simulink model "sliding_controller2"  (R2021a)
settings: Solver=ode3  StartTime=0.0  StopTime=inf  FixedStep=.001  RelTol=1e-3  EnableMultiTasking=on
model workspace (MAT data in the model file):
  SL_ROS_VariableLengthArrays_MaxSizes.CommonInfo.ArrayTruncateAction = 'EmitWarning'
  SL_ROS_VariableLengthArrays_MaxSizes.MsgTypeMap = containers.Map
  SL_ROS_VariableLengthArrays_MaxSizes.MsgTypeMap.serialization.keys = {'ambf_walker/DesiredJoints', 'rbdl_server/RBDLInverseDynamicsRequest', 'rbdl_server/RBDLInverseDynamicsResponse', 'sensor_msgs/JointState', 'std_msgs/Float32MultiArray', 'std_msgs/Float64MultiArray'}
  SL_ROS_VariableLengthArrays_MaxSizes.MsgTypeMap.serialization.values{1}(1).PropertyName = 'Controller'
  SL_ROS_VariableLengthArrays_MaxSizes.MsgTypeMap.serialization.values{1}(1).DataType = 'uint8'
  SL_ROS_VariableLengthArrays_MaxSizes.MsgTypeMap.serialization.values{1}(1).MaxLength = 8
  SL_ROS_VariableLengthArrays_MaxSizes.MsgTypeMap.serialization.values{1}(2).PropertyName = 'Other'
  SL_ROS_VariableLengthArrays_MaxSizes.MsgTypeMap.serialization.values{1}(2).DataType = 'double'
  SL_ROS_VariableLengthArrays_MaxSizes.MsgTypeMap.serialization.values{1}(2).MaxLength = 7
  SL_ROS_VariableLengthArrays_MaxSizes.MsgTypeMap.serialization.values{1}(3).PropertyName = 'Q'
  SL_ROS_VariableLengthArrays_MaxSizes.MsgTypeMap.serialization.values{1}(3).DataType = 'double'
  SL_ROS_VariableLengthArrays_MaxSizes.MsgTypeMap.serialization.values{1}(3).MaxLength = 7
  SL_ROS_VariableLengthArrays_MaxSizes.MsgTypeMap.serialization.values{1}(4).PropertyName = 'Qd'
  SL_ROS_VariableLengthArrays_MaxSizes.MsgTypeMap.serialization.values{1}(4).DataType = 'double'
  SL_ROS_VariableLengthArrays_MaxSizes.MsgTypeMap.serialization.values{1}(4).MaxLength = 7
  SL_ROS_VariableLengthArrays_MaxSizes.MsgTypeMap.serialization.values{1}(5).PropertyName = 'Qdd'
  SL_ROS_VariableLengthArrays_MaxSizes.MsgTypeMap.serialization.values{1}(5).DataType = 'double'
  SL_ROS_VariableLengthArrays_MaxSizes.MsgTypeMap.serialization.values{1}(5).MaxLength = 7
  SL_ROS_VariableLengthArrays_MaxSizes.MsgTypeMap.serialization.values{2}(1).PropertyName = 'ModelName'
  SL_ROS_VariableLengthArrays_MaxSizes.MsgTypeMap.serialization.values{2}(1).DataType = 'uint8'
  SL_ROS_VariableLengthArrays_MaxSizes.MsgTypeMap.serialization.values{2}(1).MaxLength = 4
  SL_ROS_VariableLengthArrays_MaxSizes.MsgTypeMap.serialization.values{2}(2).PropertyName = 'Q'
  SL_ROS_VariableLengthArrays_MaxSizes.MsgTypeMap.serialization.values{2}(2).DataType = 'double'
  SL_ROS_VariableLengthArrays_MaxSizes.MsgTypeMap.serialization.values{2}(2).MaxLength = 7
  SL_ROS_VariableLengthArrays_MaxSizes.MsgTypeMap.serialization.values{2}(3).PropertyName = 'Qd'
  SL_ROS_VariableLengthArrays_MaxSizes.MsgTypeMap.serialization.values{2}(3).DataType = 'double'
  SL_ROS_VariableLengthArrays_MaxSizes.MsgTypeMap.serialization.values{2}(3).MaxLength = 7
  SL_ROS_VariableLengthArrays_MaxSizes.MsgTypeMap.serialization.values{2}(4).PropertyName = 'Qdd'
  SL_ROS_VariableLengthArrays_MaxSizes.MsgTypeMap.serialization.values{2}(4).DataType = 'double'
  SL_ROS_VariableLengthArrays_MaxSizes.MsgTypeMap.serialization.values{2}(4).MaxLength = 7
  SL_ROS_VariableLengthArrays_MaxSizes.MsgTypeMap.serialization.values{3}.PropertyName = 'Tau'
  SL_ROS_VariableLengthArrays_MaxSizes.MsgTypeMap.serialization.values{3}.DataType = 'double'
  SL_ROS_VariableLengthArrays_MaxSizes.MsgTypeMap.serialization.values{3}.MaxLength = 7
  SL_ROS_VariableLengthArrays_MaxSizes.MsgTypeMap.serialization.values{4}(1).PropertyName = 'Effort'
  SL_ROS_VariableLengthArrays_MaxSizes.MsgTypeMap.serialization.values{4}(1).DataType = 'double'
  SL_ROS_VariableLengthArrays_MaxSizes.MsgTypeMap.serialization.values{4}(1).MaxLength = 7
  SL_ROS_VariableLengthArrays_MaxSizes.MsgTypeMap.serialization.values{4}(2).PropertyName = 'Name'
  SL_ROS_VariableLengthArrays_MaxSizes.MsgTypeMap.serialization.values{4}(2).DataType = 'std_msgs/String'
  SL_ROS_VariableLengthArrays_MaxSizes.MsgTypeMap.serialization.values{4}(2).MaxLength = 16
  SL_ROS_VariableLengthArrays_MaxSizes.MsgTypeMap.serialization.values{4}(3).PropertyName = 'Position'
  SL_ROS_VariableLengthArrays_MaxSizes.MsgTypeMap.serialization.values{4}(3).DataType = 'double'
  SL_ROS_VariableLengthArrays_MaxSizes.MsgTypeMap.serialization.values{4}(3).MaxLength = 7
  SL_ROS_VariableLengthArrays_MaxSizes.MsgTypeMap.serialization.values{4}(4).PropertyName = 'Velocity'
  SL_ROS_VariableLengthArrays_MaxSizes.MsgTypeMap.serialization.values{4}(4).DataType = 'double'
  SL_ROS_VariableLengthArrays_MaxSizes.MsgTypeMap.serialization.values{4}(4).MaxLength = 7
  SL_ROS_VariableLengthArrays_MaxSizes.MsgTypeMap.serialization.values{5}.PropertyName = 'Data'
  SL_ROS_VariableLengthArrays_MaxSizes.MsgTypeMap.serialization.values{5}.DataType = 'single'
  SL_ROS_VariableLengthArrays_MaxSizes.MsgTypeMap.serialization.values{5}.MaxLength = 7
  SL_ROS_VariableLengthArrays_MaxSizes.MsgTypeMap.serialization.values{6}.PropertyName = 'Data'
  SL_ROS_VariableLengthArrays_MaxSizes.MsgTypeMap.serialization.values{6}.DataType = 'double'
  SL_ROS_VariableLengthArrays_MaxSizes.MsgTypeMap.serialization.values{6}.MaxLength = 7
  SL_ROS_VariableLengthArrays_MaxSizes.MsgTypeMap.serialization.uniformity = 0
  SL_ROS_VariableLengthArrays_MaxSizes.MsgTypeMap.serialization.keyType = 'char'
  SL_ROS_VariableLengthArrays_MaxSizes.MsgTypeMap.serialization.valueType = 'any'
values from neighbouring files (symbols this model uses):
  alpha = [15,15]    [init_with_opt_gains.m]    (also in trying01.m = params.all_cost_parameters(5,1).Value; trying02.m = params.all_cost_parameters(5,1).Value)
  beta = zeros(7,1) + params.all_cost_parameters(6,1).Value(1)    [init_with_opt_gains.m]    (also in trying01.m; trying02.m = zeros(6,1) + params.all_cost_parameters(6,1).Value(1))
  Bn0 = [Bn0_hip Bn0_knee Bn0_ankle Bn0_hip Bn0_knee Bn0_ankle 0.0]    [init_with_opt_gains.m]    (also in sliding_controller_init.m = 50; trying01.m; trying02.m = [Bn0_hip Bn0_knee Bn0_ankle Bn0_hip Bn0_knee Bn0_ankle ])
  Bp0 = [Bp0_hip Bp0_knee Bp0_ankle Bp0_hip Bp0_knee Bp0_ankle 0.0]    [init_with_opt_gains.m]    (also in sliding_controller_init.m = 50; trying01.m; trying02.m = [Bp0_hip Bp0_knee Bp0_ankle Bp0_hip Bp0_knee Bp0_ankle ])
  dampener = 0.01*eye(2)    [init_with_opt_gains.m]    (also in sliding_controller_init.m = 100*eye(2); trying01.m = [30, 0; 0, 30]; trying02.m = [0.30, 0; 0, 0.30])
  Dm1 = 30*eye(7)    [init_with_opt_gains.m]    (also in sliding_controller_init.m; trying01.m = [Dm_hip, 0.0, 0.0, 0.0, 0.0, 0.0,0; trying02.m = [101.7013888888889 0 0 0 0 0)
  exo_sat = 150    [init_with_opt_gains.m]    (also in sliding_controller_init.m = 50; trying01.m = 250; trying02.m = 30)
  gamma = [15,15]    [init_with_opt_gains.m]    (also in trying01.m = params.all_cost_parameters(7,1).Value; trying02.m = params.all_cost_parameters(7,1).Value)
  human_sat = 30    [init_with_opt_gains.m]    (also in sliding_controller_init.m = 10; trying01.m = 0; trying02.m = 20)
  invMd = inv(Md)    [init_with_opt_gains.m]    (also in sliding_controller_init.m; trying01.m; trying02.m)
  Km1 = 30*eye(7)    [init_with_opt_gains.m]    (also in sliding_controller_init.m; trying01.m = [Km_hip, 0.0, 0.0, 0.0, 0.0, 0.0,0; trying02.m = [6120.116528948097 0 0 0 0 0)
  Kn0 = [Kn0_hip Kn0_knee Kn0_ankle Kn0_hip Kn0_knee Kn0_ankle 0.0]    [init_with_opt_gains.m]    (also in sliding_controller_init.m = 50*eye(7); trying01.m; trying02.m = [Kn0_hip Kn0_knee Kn0_ankle Kn0_hip Kn0_knee Kn0_ankle ])
  Kp0 = [Kp0_hip Kp0_knee Kp_ankle Kp0_hip Kp0_knee Kp0_ankle 0.0]    [init_with_opt_gains.m]    (also in sliding_controller_init.m = 50*eye(7); trying01.m = [Kp0_hip Kp0_knee Kp0_ankle Kp0_hip Kp0_knee Kp0_ankle 0.0]; trying02.m = [Kp0_hip Kp0_knee Kp0_ankle Kp0_hip Kp0_knee Kp0_ankle ])
  lambda2 = [lambda_hip, 0, 0, 0, 0, 0,0 ... (first row only)    [init_with_opt_gains.m]    (also in sliding_controller_init.m = eye(7); trying01.m; trying02.m = [lambda_hip, 0, 0, 0, 0, 0)
  rho2 = [rho_hip, 0.0, 0.0, 0.0, 0.0, 0.0,0 ... (first row only)    [init_with_opt_gains.m]    (also in sliding_controller_init.m = 200*eye(7); trying01.m; trying02.m = [rho_hip, 0.0, 0.0, 0.0, 0.0, 0.0)
  spring = 0.01*eye(2)    [init_with_opt_gains.m]    (also in sliding_controller_init.m = 100*eye(2); trying01.m = [30, 0; 0, 30]; trying02.m = [0.30, 0; 0, 0.30])
undefined symbols (not defined in the file or in its folder): Effort, Header, l, mh, Position, Q, Qd, Qdd, Velocity
libraries: robotlib x24
settings Model: SimulationMode=external  TunableVars=Bd,Bn0,Bp0,Dm1,Kd,Kd_e,Ked,Kem,Km1,Kn0,Kp0,Kp_e,Md,alpha_n,alpha_p,beta_n,beta_p,dampener,exo_sat,invMd,l1,l2,lambda2,myQ,myR,rho2,sat,spring  TunableVarsStorageClass=ExportedGlobal,ExportedGlobal,ExportedGlobal,ExportedGlobal,ExportedGlobal,ExportedGlobal,ExportedGlobal,ExportedGlobal,ExportedGlobal,ExportedGlobal,ExportedGlobal,ExportedGlobal,ExportedGlobal,ExportedGlobal,ExportedGlobal,ExportedGlobal,ExportedGlobal,ExportedGlobal,ExportedGlobal,ExportedGlobal,ExportedGlobal,ExportedGlobal,ExportedGlobal,ExportedGlobal,ExportedGlobal,ExportedGlobal,Auto,Auto  TunableVarsTypeQualifier=,,,,,,,,,,,,,,,,,,,,,,,,,,,  Creator=nathanielgoldfarb  LastModifiedBy=nathanielgoldfarb
settings OptimizationCC: EnhancedBackFolding=on  PassReuseOutputArgsAs=Individual arguments  ZeroExternalMemoryAtStartup=off  ZeroInternalMemoryAtStartup=off  InitFltsAndDblsToZero=on  MaxStackSize=64  OptimizeBlockOrder=speed  DifferentSizesBufferReuse=on  OptimizationCustomize=off  EfficientTunableParamExpr=on
settings DebuggingCC: ParameterTunabilityLossMsg=error
settings HardwareCC: ProdBitPerPointer=32  ProdBitPerSizeT=32  ProdBitPerPtrDiffT=32  ProdLargestAtomicFloat=None  ProdIntDivRoundTo=Undefined  ProdEndianess=Unspecified  ProdWordSize=32  ProdHWDeviceType=Generic->Unspecified (assume 32-bit Generic)  TargetLongLongMode=on
settings SFSimCC: MATLABDynamicMemAlloc=off  SimTargetLang=C++  GPUAcceleration=on  SimDLTargetLibrary=cudnn
settings RTWCC: SystemTargetFile=ert.tlc  HardwareBoard=Robot Operating System (ROS)  TLCOptions="-aInlineSetEventsForThisBaseRateFcn=TLC_FALSE -aSuppressMultiTaskScheduler=TLC_FALSE  -aRateBasedStepFcn=0"  TemplateMakefile=ert_default_tmf  GenerateReport=on  Toolchain=Catkin  LaunchReport=on  TargetLang=C++  GenerateCodeMetricsReport=on
settings CodeAppCC: ForceParamTrailComments=on  IgnoreCustomStorageClasses=off  OperatorAnnotations=on  SimulinkDataObjDesc=on  SFDataObjDesc=on  InsertBlockDesc=on
settings ERTTargetCC: CodeInterfacePackaging=C++ class  SupportContinuousTime=on  SupportNonInlinedSFcns=on  SupportVariableSizeSignals=on  RootIOFormat=Structure reference

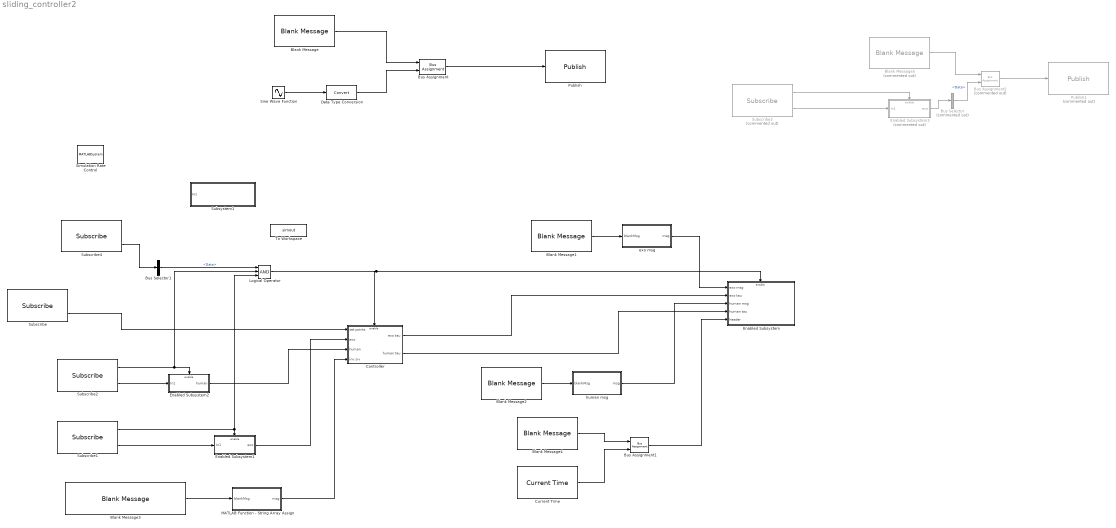
== system sliding_controller2 ==
  Blank Message : robotlib/Blank Message  messageClass=Message  entityType=std_msgs/Float32  messageType=std_msgs/Float32  SampleTime=-1  legacyBusStruct=off
  Blank Message1 : robotlib/Blank Message  messageClass=Message  entityType=sensor_msgs/JointState  messageType=sensor_msgs/JointState  SampleTime=inf  legacyBusStruct=off
  Blank Message2 : robotlib/Blank Message  messageClass=Message  entityType=sensor_msgs/JointState  messageType=sensor_msgs/JointState  SampleTime=inf  legacyBusStruct=off
  Blank Message3 : robotlib/Blank Message  messageClass=Service Request  entityType=rbdl_server/RBDLInverseDynamics  messageType=rbdl_server/RBDLInverseDynamicsRequest  SampleTime=inf  legacyBusStruct=off
  Blank Message4 : robotlib/Blank Message  messageClass=Message  entityType=std_msgs/Header  messageType=std_msgs/Header  SampleTime=inf  legacyBusStruct=off
  Blank Message5 : robotlib/Blank Message  Commented=on  messageClass=Message  entityType=std_msgs/Bool  messageType=std_msgs/Bool  SampleTime=inf  legacyBusStruct=off
  Bus Assignment : BusAssignment  AssignedSignals=Data
  Bus Assignment1 : BusAssignment  AssignedSignals=Stamp
  Bus Assignment2 : BusAssignment  Commented=on  AssignedSignals=Data
  Bus Selector : BusSelector  Commented=on  OutputSignals=Data
  Bus Selector1 : BusSelector  OutputSignals=Data
  Controller : Subsystem  TreatAsAtomicUnit=on
  Current Time : robotlib/Current Time  OutputFormat=bus  SampleTime=-1  ModelName=sliding_controller2
      settings: SourceProductBaseCode=RR
  Data Type Conversion : DataTypeConversion
  Enabled Subsystem : Subsystem  TreatAsAtomicUnit=on
  Enabled Subsystem1 : Subsystem  TreatAsAtomicUnit=on
  Enabled Subsystem2 : Subsystem  TreatAsAtomicUnit=on
  Enabled Subsystem3 : Subsystem  Commented=on  TreatAsAtomicUnit=on
  Logical Operator : Logic  Inputs=3  AllPortsSameDT=off  OutDataTypeStr=boolean
  MATLAB Function - String Array Assign : MATLAB Function  TreatAsAtomicUnit=on
  Publish : robotlib/Publish  topicSource=Specify your own  topic=/sin_wave  messageType=std_msgs/Float32  legacyBusStruct=off  messageQueueLength=1
  Publish1 : robotlib/Publish  Commented=on  topicSource=Specify your own  topic=/my_topic  messageType=std_msgs/Bool  legacyBusStruct=off  messageQueueLength=1
  Simulation Rate Control : MATLABSystem  System=ExampleHelperSimulationRateControl  SampleTime=0.001
      mask Type: ExampleHelperSimulationRateControl
      mask Display:
      | disp('Rate Control');
      | port_label('output',1,'r');
  Sine Wave Function : Sin  SampleTime=0
  Subscribe : robotlib/Subscribe  topicSource=Select from ROS network  topic=/exosimulink_set_points  messageType=ambf_walker/DesiredJoints  SampleTime=-1  legacyBusStruct=off  messageQueueLength=1
  Subscribe1 : robotlib/Subscribe  topicSource=Select from ROS network  topic=/exo_jointstate  messageType=sensor_msgs/JointState  SampleTime=-1  legacyBusStruct=off  messageQueueLength=1
  Subscribe2 : robotlib/Subscribe  topicSource=Select from ROS network  topic=/human_jointstate  messageType=sensor_msgs/JointState  SampleTime=-1  legacyBusStruct=off  messageQueueLength=1
  Subscribe3 : robotlib/Subscribe  Commented=on  topicSource=Specify your own  topic=/start  messageType=std_msgs/Bool  SampleTime=-1  legacyBusStruct=off  messageQueueLength=1
  Subscribe4 : robotlib/Subscribe  topicSource=Specify your own  topic=/start_sim  messageType=std_msgs/Bool  SampleTime=-1  legacyBusStruct=off  messageQueueLength=1
  Subsystem1 : Subsystem
  To Workspace : ToWorkspace  VariableName=simout  SampleTime=-1
      settings: Save2DSignal=2-D array (concatenate along first dimension)
  exo msg : MATLAB Function  TreatAsAtomicUnit=on
  human msg : MATLAB Function  TreatAsAtomicUnit=on
  wires:
  Data Type Conversion/1 -> Bus Assignment/2
  Blank Message/1 -> Bus Assignment/1
  Sine Wave Function/1 -> Data Type Conversion/1
  Bus Assignment/1 -> Publish/1
  human msg/1(msg) -> Enabled Subsystem/3(human msg)
  Controller/1(exo tau) -> Enabled Subsystem/2(exo tau)
  Blank Message2/1 -> human msg/1(blankMsg)
  Enabled Subsystem2/1(human) -> Controller/3(human)
  Blank Message1/1 -> exo msg/1(blankMsg)
  MATLAB Function - String Array Assign/1(msg) -> Controller/4(inv srv)
  Blank Message3/1 -> MATLAB Function - String Array Assign/1(blankMsg)
  Controller/2(human tau) -> Enabled Subsystem/4(human tau)
  Subscribe2/2 -> Enabled Subsystem2/1(In1)
  Subscribe1/2 -> Enabled Subsystem1/1(In1)
  Enabled Subsystem1/1(exo) -> Controller/2(exo)
  exo msg/1(msg) -> Enabled Subsystem/1(exo msg)
  Subscribe2/1 -> Logical Operator/2, Enabled Subsystem2/Enable
  Subscribe1/1 -> Enabled Subsystem1/Enable, Logical Operator/3
  Blank Message4/1 -> Bus Assignment1/1
  Current Time/1 -> Bus Assignment1/2
  Bus Assignment1/1 -> Enabled Subsystem/5(header)
  Subscribe3/2 -> Enabled Subsystem3/1(In1)
  Subscribe3/1 -> Enabled Subsystem3/Enable
  Enabled Subsystem3/1(exo) -> Bus Selector/1
  Bus Selector/1 -> Bus Assignment2/2  "<Data>"
  Blank Message5/1 -> Bus Assignment2/1
  Bus Assignment2/1 -> Publish1/1
  Subscribe4/2 -> Bus Selector1/1
  Bus Selector1/1 -> Logical Operator/1  "<Data>"
  Logical Operator/1 -> Enabled Subsystem/Enable, Controller/Enable
  Subscribe/2 -> Controller/1(set points)

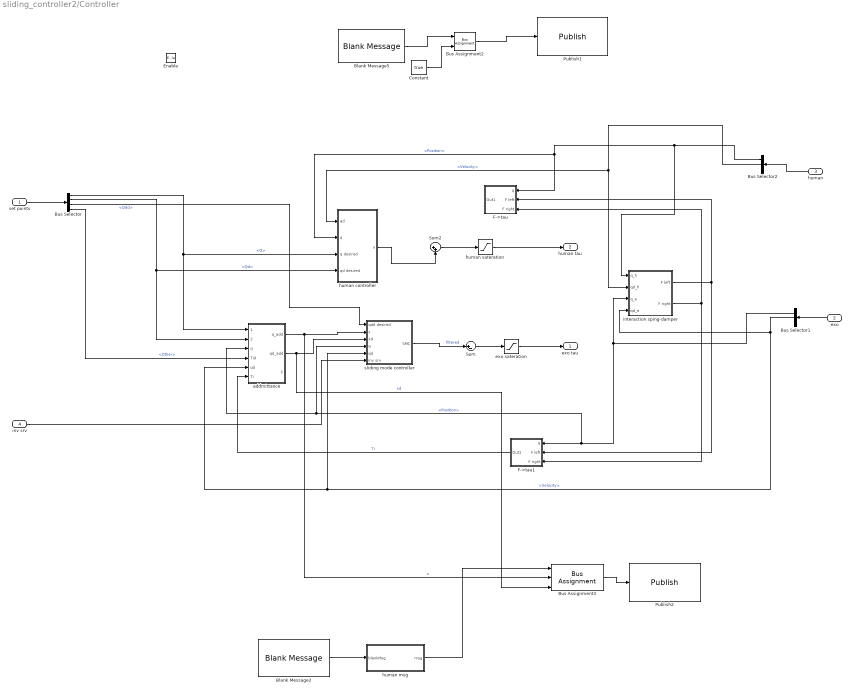
== system sliding_controller2/Controller ==
  set points : Inport
  exo : Inport  Port=2
  human : Inport  Port=3
  inv srv : Inport  Port=4
  Enable : EnablePort
  " interaction sping-damper" : Subsystem
  Blank Message2 : robotlib/Blank Message  messageClass=Message  entityType=sensor_msgs/JointState  messageType=sensor_msgs/JointState  SampleTime=inf  legacyBusStruct=off
  Blank Message5 : robotlib/Blank Message  messageClass=Message  entityType=std_msgs/Bool  messageType=std_msgs/Bool  SampleTime=inf  legacyBusStruct=off
  Bus Assignment2 : BusAssignment  AssignedSignals=Data
  Bus Assignment3 : BusAssignment  AssignedSignals=Position,Velocity
  Bus Selector : BusSelector  OutputSignals=Q,Qd,Qdd,Other
  Bus Selector1 : BusSelector  OutputSignals=Position,Velocity,Effort
  Bus Selector2 : BusSelector  OutputSignals=Position,Velocity,Effort
  Constant : Constant  Value=true  VectorParams1D=off
  F->tau : Subsystem
  F->tau1 : Subsystem
  Publish1 : robotlib/Publish  topicSource=Specify your own  topic=/my_topic  messageType=std_msgs/Bool  legacyBusStruct=off  messageQueueLength=1
  Publish2 : robotlib/Publish  topicSource=Specify your own  topic=addmittance  messageType=sensor_msgs/JointState  legacyBusStruct=off  messageQueueLength=1
  Sum : Sum  Inputs=|+-
  Sum2 : Sum  Inputs=|++
  addmittance : Subsystem
  exo sateration : Saturate  UpperLimit=exo_sat  LowerLimit=-exo_sat
  human controller : Subsystem
  human msg : MATLAB Function  TreatAsAtomicUnit=on
  human sateration : Saturate  UpperLimit=human_sat  LowerLimit=-human_sat
  sliding mode controller : Subsystem
  exo tau : Outport
  human tau : Outport  Port=2
  wires:
  Bus Selector/4 -> addmittance/4(Tid)  "<Other>"
  exo sateration/1 -> exo tau/1
  addmittance/2(qd_add) -> Bus Assignment3/3, sliding mode controller/3(xd)  "xd"
  sliding mode controller/1(SMC) -> Sum/1  "filtered"
  " interaction sping-damper"/2(F right) -> F->tau1/3(F right), F->tau/3(F right)
  set points/1 -> Bus Selector/1
  human controller/1(u) -> Sum2/2
  Bus Selector/1 -> addmittance/1(q desird), human controller/3(q desired)  "<Q>"
  " interaction sping-damper"/1(F left) -> F->tau1/2(F left), F->tau/2(F left)
  addmittance/1(q_add) -> Bus Assignment3/2, sliding mode controller/2(x)  "x"
  Bus Selector/3 -> sliding mode controller/1(qdd desired)  "<Qdd>"
  Sum/1 -> exo sateration/1
  Bus Selector/2 -> addmittance/2(qd desird), human controller/4(qd desired)  "<Qd>"
  Sum2/1 -> human sateration/1
  F->tau1/1(Out1) -> addmittance/6(Ti)  "Ti"
  Bus Selector1/1 -> addmittance/3(q), sliding mode controller/4(q), F->tau1/1(q), " interaction sping-damper"/3(q_e)  "<Position>"
  Bus Selector1/2 -> " interaction sping-damper"/4("qd_e "), addmittance/5(qd), sliding mode controller/5(qd)  "<Velocity>"
  exo/1 -> Bus Selector1/1
  Bus Selector2/1 -> " interaction sping-damper"/1(q_h), human controller/2(q), F->tau/1(q)  "<Position>"
  human/1 -> Bus Selector2/1
  Bus Selector2/2 -> " interaction sping-damper"/2(qd_h), human controller/1(qd)  "<Velocity>"
  inv srv/1 -> sliding mode controller/6(inv srv)
  Constant/1 -> Bus Assignment2/2
  Blank Message5/1 -> Bus Assignment2/1
  Bus Assignment2/1 -> Publish1/1
  human sateration/1 -> human tau/1
  Bus Assignment3/1 -> Publish2/1
  Blank Message2/1 -> human msg/1(blankMsg)
  human msg/1(msg) -> Bus Assignment3/1

== system sliding_controller2/Enabled Subsystem ==
  exo msg : Inport
  exo tau : Inport  Port=2
  human msg : Inport  Port=3
  human tau : Inport  Port=4
  header : Inport  Port=5
  Enable : EnablePort
  Bus Assignment1 : BusAssignment  AssignedSignals=Effort,Header
  Bus Assignment2 : BusAssignment  AssignedSignals=Effort,Header
  Publish1 : robotlib/Publish  topicSource=Select from ROS network  topic=/exo_simulink_torque  messageType=sensor_msgs/JointState  legacyBusStruct=off  messageQueueLength=1
  Publish2 : robotlib/Publish  topicSource=Select from ROS network  topic=/human_simulink_torque  messageType=sensor_msgs/JointState  legacyBusStruct=off  messageQueueLength=1
  wires:
  human tau/1 -> Bus Assignment2/2
  exo tau/1 -> Bus Assignment1/2
  Bus Assignment2/1 -> Publish2/1
  Bus Assignment1/1 -> Publish1/1
  exo msg/1 -> Bus Assignment1/1
  human msg/1 -> Bus Assignment2/1
  header/1 -> Bus Assignment1/3, Bus Assignment2/3

== system sliding_controller2/Enabled Subsystem1 ==
  In1 : Inport
  Enable : EnablePort
  exo : Outport
  wires:
  In1/1 -> exo/1

== system sliding_controller2/Enabled Subsystem2 ==
  In1 : Inport
  Enable : EnablePort
  human : Outport
  wires:
  In1/1 -> human/1

== system sliding_controller2/Enabled Subsystem3 ==
  In1 : Inport
  Enable : EnablePort
  exo : Outport
  wires:
  In1/1 -> exo/1

== system sliding_controller2/Subsystem1 ==
  In1 : Inport
  Constant : Constant  Value=false
  Data Type Conversion : DataTypeConversion
  If : If  IfExpression=u1 == 1
  If Action Subsystem : Subsystem  TreatAsAtomicUnit=on
  wires:
  In1/1 -> Data Type Conversion/1
  If/1 -> If Action Subsystem/Action
  Data Type Conversion/1 -> If/1
  Constant/1 -> If Action Subsystem/1(In1)

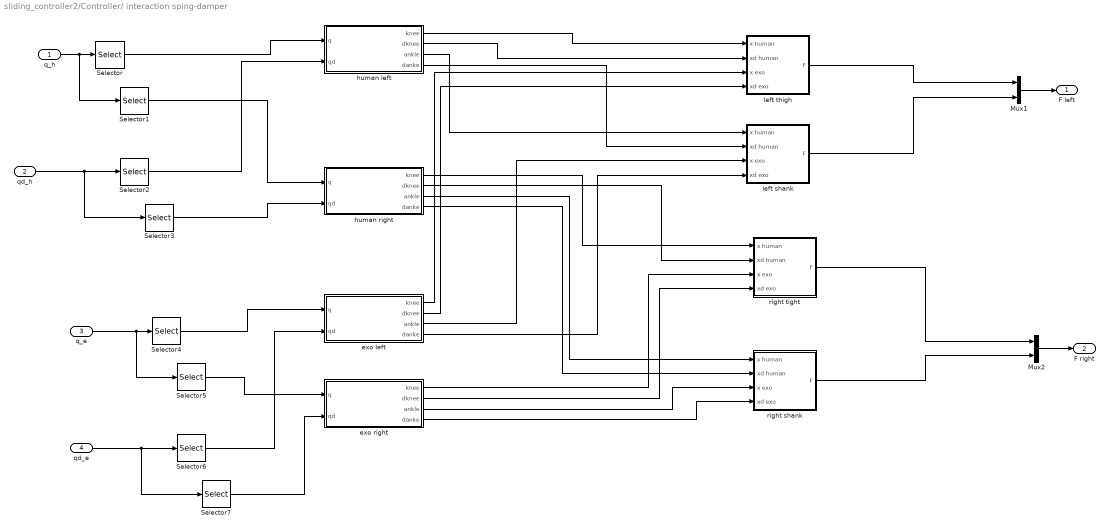
== system sliding_controller2/Controller/ interaction sping-damper ==
  q_h : Inport
  qd_h : Inport  Port=2
  q_e : Inport  Port=3
  "qd_e " : Inport  Port=4
  Mux1 : Mux  Inputs=2
  Mux2 : Mux  Inputs=2
  Selector{,2,4,6} (4 alike) : Selector  InputPortWidth=7  IndexOptions=Index vector (dialog)  Indices=[1 2]  OutputSizes=1
  Selector{1,3,5,7} (4 alike) : Selector  InputPortWidth=7  IndexOptions=Index vector (dialog)  Indices=[4 5]  OutputSizes=1
  exo left : MATLAB Function  TreatAsAtomicUnit=on
  exo right : MATLAB Function  TreatAsAtomicUnit=on
  human left : MATLAB Function  TreatAsAtomicUnit=on
  human right : MATLAB Function  TreatAsAtomicUnit=on
  left shank : Subsystem
  left thigh : Subsystem
  right shank : Subsystem
  right tight : Subsystem
  F left : Outport
  F right : Outport  Port=2
  wires:
  q_h/1 -> Selector1/1, Selector/1
  Selector/1 -> human left/1(q)
  Selector1/1 -> human right/1(q)
  Selector2/1 -> human left/2(qd)
  Selector3/1 -> human right/2(qd)
  qd_h/1 -> Selector3/1, Selector2/1
  q_e/1 -> Selector5/1, Selector4/1
  Selector4/1 -> exo left/1(q)
  Selector5/1 -> exo right/1(q)
  "qd_e "/1 -> Selector7/1, Selector6/1
  Selector7/1 -> exo right/2(qd)
  Selector6/1 -> exo left/2(qd)
  human left/1(knee) -> left thigh/1(x human)
  human left/2(dknee) -> left thigh/2("xd human ")
  human left/3(ankle) -> left shank/1(x human)
  human left/4(danke) -> left shank/2("xd human ")
  exo left/1(knee) -> left thigh/3(x exo)
  exo left/2(dknee) -> left thigh/4(xd exo)
  exo left/3(ankle) -> left shank/3(x exo)
  exo left/4(danke) -> left shank/4(xd exo)
  human right/4(danke) -> right shank/2("xd human ")
  exo right/1(knee) -> right tight/3(x exo)
  human right/1(knee) -> right tight/1(x human)
  exo right/3(ankle) -> right shank/3(x exo)
  exo right/4(danke) -> right shank/4(xd exo)
  exo right/2(dknee) -> right tight/4(xd exo)
  human right/3(ankle) -> right shank/1(x human)
  human right/2(dknee) -> right tight/2("xd human ")
  Mux1/1 -> F left/1
  left shank/1(F) -> Mux1/2
  left thigh/1(F) -> Mux1/1
  Mux2/1 -> F right/1
  right tight/1(F) -> Mux2/1
  right shank/1(F) -> Mux2/2

== system sliding_controller2/Controller/F->tau ==
  q : Inport
  F left : Inport  Port=2
  F right : Inport  Port=3
  Constant : Constant  Value=0
  Mux : Mux  Inputs=3
  Selector : Selector  InputPortWidth=7  IndexOptions=Index vector (dialog)  Indices=[1 2]  OutputSizes=1
  Selector1 : Selector  InputPortWidth=7  IndexOptions=Index vector (dialog)  Indices=[4 5]  OutputSizes=1
  Subsystem : Subsystem
  Subsystem1 : Subsystem
  Out1 : Outport
  wires:
  Subsystem/1(tau) -> Mux/1
  q/1 -> Selector1/1, Selector/1
  Selector/1 -> Subsystem/1(q)
  F left/1 -> Subsystem/2(F)
  Selector1/1 -> Subsystem1/1(q)
  F right/1 -> Subsystem1/2(F)
  Subsystem1/1(tau) -> Mux/2
  Mux/1 -> Out1/1
  Constant/1 -> Mux/3

== system sliding_controller2/Controller/F->tau1 ==
  q : Inport
  F left : Inport  Port=2
  F right : Inport  Port=3
  Constant : Constant  Value=0
  Mux : Mux  Inputs=3
  Selector : Selector  InputPortWidth=7  IndexOptions=Index vector (dialog)  Indices=[1 2]  OutputSizes=1
  Selector1 : Selector  InputPortWidth=7  IndexOptions=Index vector (dialog)  Indices=[4 5]  OutputSizes=1
  Subsystem : Subsystem
  Subsystem1 : Subsystem
  Out1 : Outport
  wires:
  Subsystem1/1(tau) -> Mux/1
  q/1 -> Selector1/1, Selector/1
  Selector/1 -> Subsystem1/1(q)
  F left/1 -> Subsystem1/2(F)
  Selector1/1 -> Subsystem/1(q)
  F right/1 -> Subsystem/2(F)
  Subsystem/1(tau) -> Mux/2
  Mux/1 -> Out1/1
  Constant/1 -> Mux/3

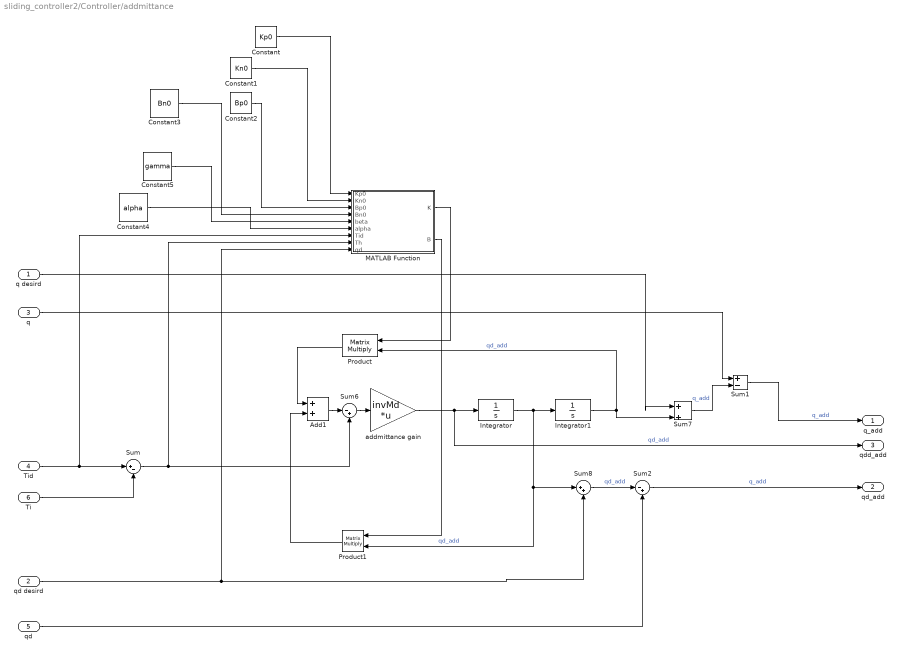
== system sliding_controller2/Controller/addmittance ==
  q desird : Inport
  qd desird : Inport  Port=2
  q : Inport  Port=3
  Tid : Inport  Port=4
  qd : Inport  Port=5
  Ti : Inport  Port=6
  Add1 : Sum
  Constant : Constant  Value=Kp0
  Constant1 : Constant  Value=Kn0
  Constant2 : Constant  Value=Bp0
  Constant3 : Constant  Value=Bn0
  Constant4 : Constant  Value=alpha
  Constant5 : Constant  Value=gamma
  Integrator : Integrator
  Integrator1 : Integrator  InitialCondition=[-0.349,-0.2,0,-0.349,-0.2,0,0]
  MATLAB Function : MATLAB Function  TreatAsAtomicUnit=on
  Product : Product  Multiplication=Matrix(*)
  Product1 : Product  Multiplication=Matrix(*)
  Sum : Sum  Inputs=|+-
  Sum1 : Sum  Inputs=|+-
  Sum2 : Sum  Inputs=|-+
  Sum6 : Sum  Inputs=|-+
  Sum7 : Sum  Inputs=|++
  Sum8 : Sum  Inputs=|++
  addmittance gain : Gain  Gain=invMd  Multiplication=Matrix(K*u)
  q_add : Outport
  qd_add : Outport  Port=2
  qdd_add : Outport  Port=3
  wires:
  Add1/1 -> Sum6/1
  qd desird/1 -> MATLAB Function/9(qd), Sum8/2
  addmittance gain/1 -> qdd_add/1, Integrator/1  "qd_add"
  Sum6/1 -> addmittance gain/1
  Product/1 -> Add1/1
  q desird/1 -> Sum7/1
  qd/1 -> Sum2/2
  Sum2/1 -> qd_add/1  "q_add"
  Sum7/1 -> Sum1/2  "q_add"
  q/1 -> Sum1/1
  Sum1/1 -> q_add/1  "q_add"
  Sum8/1 -> Sum2/1  "qd_add"
  Integrator/1 -> Product1/2, Sum8/1, Integrator1/1  "qd_add"
  Integrator1/1 -> Product/2, Sum7/2  "qd_add"
  Sum/1 -> MATLAB Function/8(Th), Sum6/2
  Tid/1 -> MATLAB Function/7(Tid), Sum/1
  Ti/1 -> Sum/2
  Product1/1 -> Add1/2
  MATLAB Function/1(K) -> Product/1
  MATLAB Function/2(B) -> Product1/1
  Constant3/1 -> MATLAB Function/4(Bn0)
  Constant4/1 -> MATLAB Function/6(alpha)
  Constant1/1 -> MATLAB Function/2(Kn0)
  Constant5/1 -> MATLAB Function/5(beta)
  Constant2/1 -> MATLAB Function/3(Bp0)
  Constant/1 -> MATLAB Function/1(Kp0)

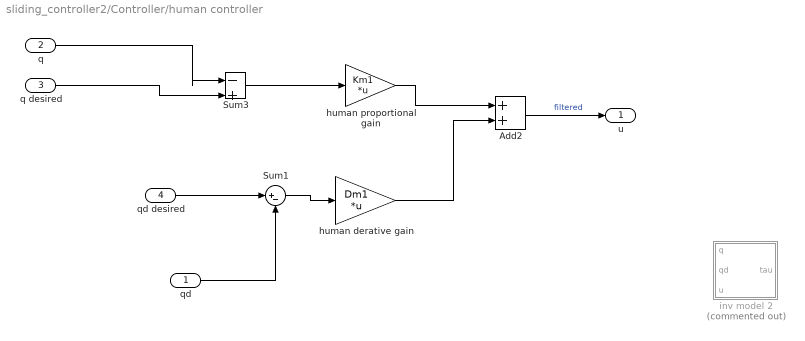
== system sliding_controller2/Controller/human controller ==
  qd : Inport
  q : Inport  Port=2
  q desired : Inport  Port=3
  qd desired : Inport  Port=4
  Add2 : Sum
  Sum1 : Sum  Inputs=|+-
  Sum3 : Sum  Inputs=|-+
  human derative gain : Gain  Gain=Dm1  Multiplication=Matrix(K*u)
  human proportional gain : Gain  Gain=Km1  Multiplication=Matrix(K*u)
  inv model 2 : Subsystem  Commented=on
  u : Outport
  wires:
  Sum1/1 -> human derative gain/1
  qd/1 -> Sum1/2
  Sum3/1 -> human proportional gain/1
  human derative gain/1 -> Add2/2
  q desired/1 -> Sum3/2
  human proportional gain/1 -> Add2/1
  qd desired/1 -> Sum1/1
  q/1 -> Sum3/1
  Add2/1 -> u/1  "filtered"

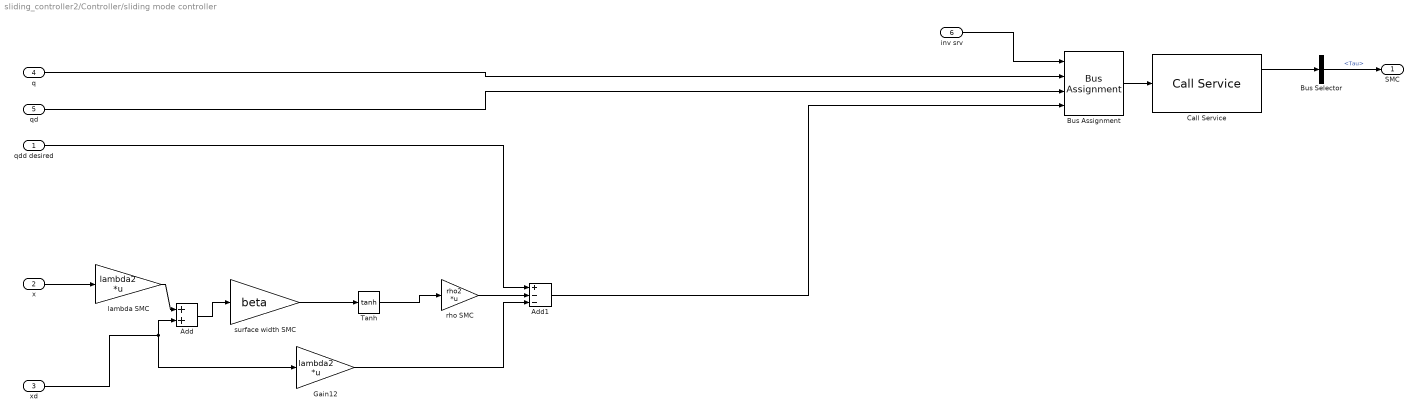
== system sliding_controller2/Controller/sliding mode controller ==
  qdd desired : Inport
  x : Inport  Port=2
  xd : Inport  Port=3
  q : Inport  Port=4
  qd : Inport  Port=5
  inv srv : Inport  Port=6
  Add : Sum
  Add1 : Sum  Inputs=+--
  Bus Assignment : BusAssignment  AssignedSignals=Q,Qd,Qdd
  Bus Selector : BusSelector  OutputSignals=Tau
  Call Service : robotlib/Call Service  topicSource=Select from ROS network  service=/InverseDynamics  serviceType=rbdl_server/RBDLInverseDynamics  connectionTimeout=1  keepPersistent=on  ShowErrorCodeOutput=on  legacyBusStruct=off
      settings: SourceProductBaseCode=RR
  Gain12 : Gain  Gain=lambda2  Multiplication=Matrix(K*u)
  Tanh : Trigonometry  Operator=tanh
  lambda SMC : Gain  Gain=lambda2  Multiplication=Matrix(K*u)
  rho SMC : Gain  Gain=rho2  Multiplication=Matrix(K*u)
  surface width SMC : Gain  Gain=beta
  SMC : Outport
  wires:
  surface width SMC/1 -> Tanh/1
  Gain12/1 -> Add1/3
  lambda SMC/1 -> Add/1
  x/1 -> lambda SMC/1
  xd/1 -> Add/2, Gain12/1
  Add/1 -> surface width SMC/1
  rho SMC/1 -> Add1/2
  qdd desired/1 -> Add1/1
  Tanh/1 -> rho SMC/1
  q/1 -> Bus Assignment/2
  qd/1 -> Bus Assignment/3
  Bus Assignment/1 -> Call Service/1
  Call Service/1 -> Bus Selector/1
  inv srv/1 -> Bus Assignment/1
  Bus Selector/1 -> SMC/1  "<Tau>"
  Add1/1 -> Bus Assignment/4

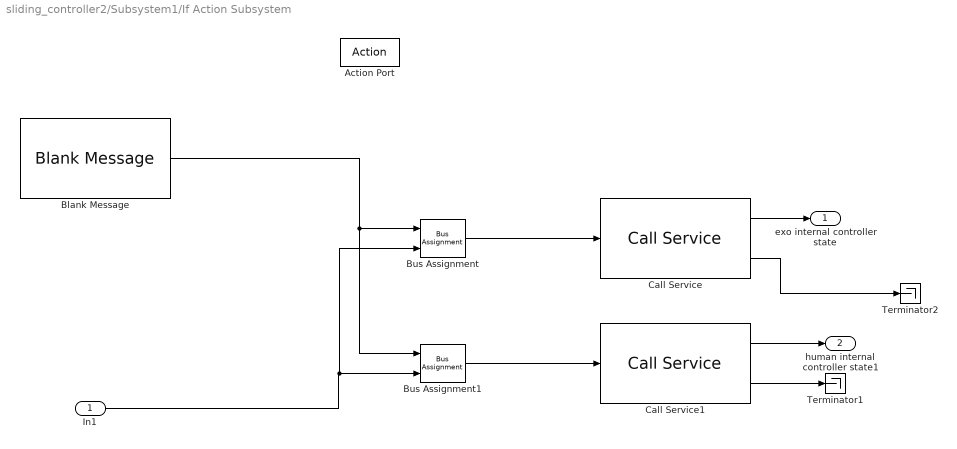
== system sliding_controller2/Subsystem1/If Action Subsystem ==
  In1 : Inport
  Action Port : ActionPort  ActionPortLabel=if(u1 == 1)
  Blank Message : robotlib/Blank Message  messageClass=Service Request  entityType=std_srvs/SetBool  messageType=std_srvs/SetBoolRequest  SampleTime=inf  legacyBusStruct=off
  Bus Assignment : BusAssignment  AssignedSignals=Data
  Bus Assignment1 : BusAssignment  AssignedSignals=Data
  Call Service : robotlib/Call Service  topicSource=Select from ROS network  service=/exo_controller_onoff  serviceType=std_srvs/SetBool  connectionTimeout=5  keepPersistent=on  ShowErrorCodeOutput=on  legacyBusStruct=off
      settings: SourceProductBaseCode=RR
  Call Service1 : robotlib/Call Service  topicSource=Select from ROS network  service=/human_controller_onoff  serviceType=std_srvs/SetBool  connectionTimeout=5  keepPersistent=on  ShowErrorCodeOutput=on  legacyBusStruct=off
      settings: SourceProductBaseCode=RR
  Terminator1 : Terminator
  Terminator2 : Terminator
  exo internal controller state : Outport
  human internal controller state1 : Outport  Port=2
  wires:
  In1/1 -> Bus Assignment/2, Bus Assignment1/2
  Bus Assignment1/1 -> Call Service1/1
  Call Service/1 -> exo internal controller state/1
  Bus Assignment/1 -> Call Service/1
  Call Service/2 -> Terminator2/1
  Blank Message/1 -> Bus Assignment1/1, Bus Assignment/1
  Call Service1/1 -> human internal controller state1/1
  Call Service1/2 -> Terminator1/1

== system sliding_controller2/Controller/ interaction sping-damper/left shank ==
  x human : Inport
  "xd human " : Inport  Port=2
  x exo : Inport  Port=3
  xd exo : Inport  Port=4
  Subtract : Sum  Inputs=-+
  Subtract1 : Sum  Inputs=-+
  Subtract2 : Sum
  dampener left shank : Gain  Gain=dampener  Multiplication=Matrix(K*u)
  spring left shank : Gain  Gain=spring  Multiplication=Matrix(K*u)
  F : Outport
  wires:
  Subtract2/1 -> F/1
  xd exo/1 -> Subtract1/2
  dampener left shank/1 -> Subtract2/2
  Subtract/1 -> spring left shank/1
  Subtract1/1 -> dampener left shank/1
  x exo/1 -> Subtract/2
  x human/1 -> Subtract/1
  "xd human "/1 -> Subtract1/1
  spring left shank/1 -> Subtract2/1

== system sliding_controller2/Controller/ interaction sping-damper/left thigh ==
  x human : Inport
  "xd human " : Inport  Port=2
  x exo : Inport  Port=3
  xd exo : Inport  Port=4
  Subtract : Sum  Inputs=-+
  Subtract1 : Sum  Inputs=-+
  Subtract2 : Sum
  dampener left thigh : Gain  Gain=dampener  Multiplication=Matrix(K*u)
  spring left thigh : Gain  Gain=spring  Multiplication=Matrix(K*u)
  F : Outport
  wires:
  Subtract2/1 -> F/1
  xd exo/1 -> Subtract1/2
  dampener left thigh/1 -> Subtract2/2
  Subtract/1 -> spring left thigh/1
  Subtract1/1 -> dampener left thigh/1
  x exo/1 -> Subtract/2
  x human/1 -> Subtract/1
  "xd human "/1 -> Subtract1/1
  spring left thigh/1 -> Subtract2/1

== system sliding_controller2/Controller/ interaction sping-damper/right shank ==
  x human : Inport
  "xd human " : Inport  Port=2
  x exo : Inport  Port=3
  xd exo : Inport  Port=4
  Subtract : Sum  Inputs=-+
  Subtract1 : Sum  Inputs=-+
  Subtract2 : Sum
  dampener right shank : Gain  Gain=dampener  Multiplication=Matrix(K*u)
  spring right thigh : Gain  Gain=spring  Multiplication=Matrix(K*u)
  F : Outport
  wires:
  Subtract2/1 -> F/1
  xd exo/1 -> Subtract1/2
  dampener right shank/1 -> Subtract2/2
  Subtract/1 -> spring right thigh/1
  Subtract1/1 -> dampener right shank/1
  x exo/1 -> Subtract/2
  x human/1 -> Subtract/1
  "xd human "/1 -> Subtract1/1
  spring right thigh/1 -> Subtract2/1

== system sliding_controller2/Controller/ interaction sping-damper/right tight ==
  x human : Inport
  "xd human " : Inport  Port=2
  x exo : Inport  Port=3
  xd exo : Inport  Port=4
  Subtract : Sum  Inputs=-+
  Subtract1 : Sum  Inputs=-+
  Subtract2 : Sum
  dampener right shank : Gain  Gain=dampener  Multiplication=Matrix(K*u)
  spring right thigh : Gain  Gain=spring  Multiplication=Matrix(K*u)
  F : Outport
  wires:
  Subtract2/1 -> F/1
  xd exo/1 -> Subtract1/2
  dampener right shank/1 -> Subtract2/2
  Subtract/1 -> spring right thigh/1
  Subtract1/1 -> dampener right shank/1
  x exo/1 -> Subtract/2
  x human/1 -> Subtract/1
  "xd human "/1 -> Subtract1/1
  spring right thigh/1 -> Subtract2/1

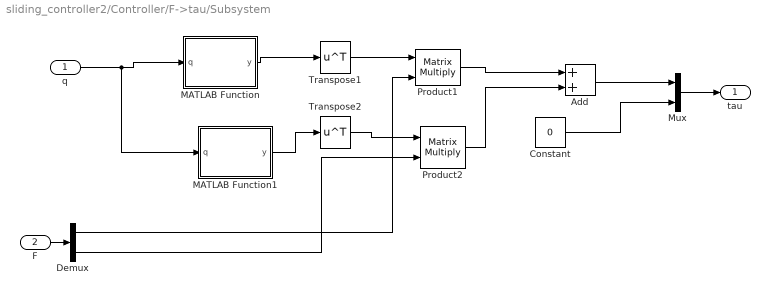
== system sliding_controller2/Controller/F->tau/Subsystem ==
  q : Inport
  F : Inport  Port=2
  Add : Sum
  Constant : Constant  Value=0
  Demux : Demux  Outputs=2
  MATLAB Function : MATLAB Function  TreatAsAtomicUnit=on
  MATLAB Function1 : MATLAB Function  TreatAsAtomicUnit=on
  Mux : Mux  Inputs=2
  Product1 : Product  Multiplication=Matrix(*)
  Product2 : Product  Multiplication=Matrix(*)
  Transpose1 : Math  Operator=transpose  SaturateOnIntegerOverflow=on
  Transpose2 : Math  Operator=transpose  SaturateOnIntegerOverflow=on
  tau : Outport
  wires:
  MATLAB Function1/1(y) -> Transpose2/1
  Transpose2/1 -> Product2/1
  Product1/1 -> Add/1
  F/1 -> Demux/1
  Product2/1 -> Add/2
  Transpose1/1 -> Product1/1
  MATLAB Function/1(y) -> Transpose1/1
  q/1 -> MATLAB Function1/1(q), MATLAB Function/1(q)
  Demux/2 -> Product2/2
  Demux/1 -> Product1/2
  Mux/1 -> tau/1
  Add/1 -> Mux/1
  Constant/1 -> Mux/2

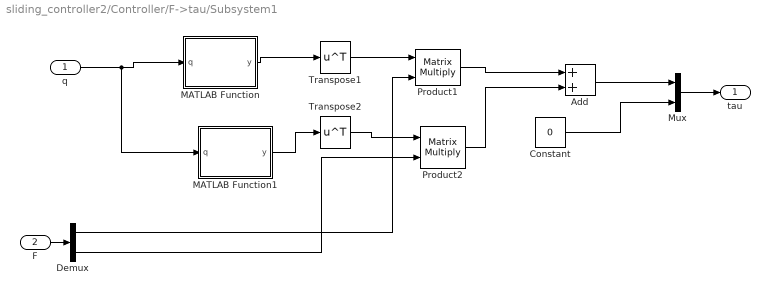
== system sliding_controller2/Controller/F->tau/Subsystem1 ==
  q : Inport
  F : Inport  Port=2
  Add : Sum
  Constant : Constant  Value=0
  Demux : Demux  Outputs=2
  MATLAB Function : MATLAB Function  TreatAsAtomicUnit=on
  MATLAB Function1 : MATLAB Function  TreatAsAtomicUnit=on
  Mux : Mux  Inputs=2
  Product1 : Product  Multiplication=Matrix(*)
  Product2 : Product  Multiplication=Matrix(*)
  Transpose1 : Math  Operator=transpose  SaturateOnIntegerOverflow=on
  Transpose2 : Math  Operator=transpose  SaturateOnIntegerOverflow=on
  tau : Outport
  wires:
  MATLAB Function1/1(y) -> Transpose2/1
  Transpose2/1 -> Product2/1
  Product1/1 -> Add/1
  F/1 -> Demux/1
  Product2/1 -> Add/2
  Transpose1/1 -> Product1/1
  MATLAB Function/1(y) -> Transpose1/1
  q/1 -> MATLAB Function1/1(q), MATLAB Function/1(q)
  Demux/2 -> Product2/2
  Demux/1 -> Product1/2
  Mux/1 -> tau/1
  Add/1 -> Mux/1
  Constant/1 -> Mux/2

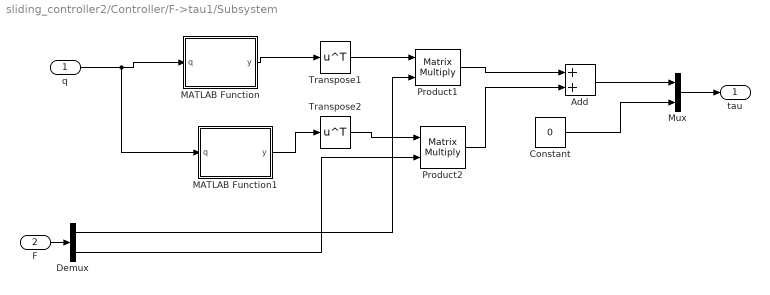
== system sliding_controller2/Controller/F->tau1/Subsystem ==
  q : Inport
  F : Inport  Port=2
  Add : Sum
  Constant : Constant  Value=0
  Demux : Demux  Outputs=2
  MATLAB Function : MATLAB Function  TreatAsAtomicUnit=on
  MATLAB Function1 : MATLAB Function  TreatAsAtomicUnit=on
  Mux : Mux  Inputs=2
  Product1 : Product  Multiplication=Matrix(*)
  Product2 : Product  Multiplication=Matrix(*)
  Transpose1 : Math  Operator=transpose  SaturateOnIntegerOverflow=on
  Transpose2 : Math  Operator=transpose  SaturateOnIntegerOverflow=on
  tau : Outport
  wires:
  MATLAB Function1/1(y) -> Transpose2/1
  Transpose2/1 -> Product2/1
  Product1/1 -> Add/1
  F/1 -> Demux/1
  Product2/1 -> Add/2
  Transpose1/1 -> Product1/1
  MATLAB Function/1(y) -> Transpose1/1
  q/1 -> MATLAB Function1/1(q), MATLAB Function/1(q)
  Demux/2 -> Product2/2
  Demux/1 -> Product1/2
  Mux/1 -> tau/1
  Add/1 -> Mux/1
  Constant/1 -> Mux/2

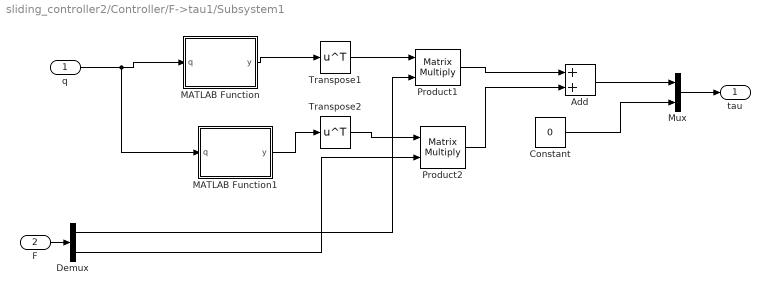
== system sliding_controller2/Controller/F->tau1/Subsystem1 ==
  q : Inport
  F : Inport  Port=2
  Add : Sum
  Constant : Constant  Value=0
  Demux : Demux  Outputs=2
  MATLAB Function : MATLAB Function  TreatAsAtomicUnit=on
  MATLAB Function1 : MATLAB Function  TreatAsAtomicUnit=on
  Mux : Mux  Inputs=2
  Product1 : Product  Multiplication=Matrix(*)
  Product2 : Product  Multiplication=Matrix(*)
  Transpose1 : Math  Operator=transpose  SaturateOnIntegerOverflow=on
  Transpose2 : Math  Operator=transpose  SaturateOnIntegerOverflow=on
  tau : Outport
  wires:
  MATLAB Function1/1(y) -> Transpose2/1
  Transpose2/1 -> Product2/1
  Product1/1 -> Add/1
  F/1 -> Demux/1
  Product2/1 -> Add/2
  Transpose1/1 -> Product1/1
  MATLAB Function/1(y) -> Transpose1/1
  q/1 -> MATLAB Function1/1(q), MATLAB Function/1(q)
  Demux/2 -> Product2/2
  Demux/1 -> Product1/2
  Mux/1 -> tau/1
  Add/1 -> Mux/1
  Constant/1 -> Mux/2

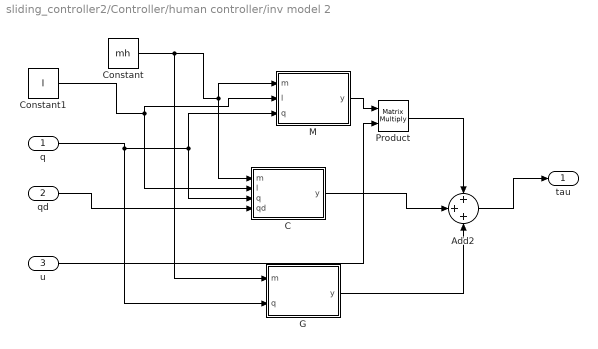
== system sliding_controller2/Controller/human controller/inv model 2 ==
  q : Inport
  qd : Inport  Port=2
  "u " : Inport  Port=3
  Add2 : Sum  Inputs=+++
  C : MATLAB Function  TreatAsAtomicUnit=on
  Constant : Constant  Value=mh
  Constant1 : Constant  Value=l
  G : MATLAB Function  TreatAsAtomicUnit=on
  M : MATLAB Function  TreatAsAtomicUnit=on
  Product : Product  Multiplication=Matrix(*)
  "tau " : Outport
  wires:
  Constant1/1 -> C/2(l), M/2(l)
  Constant/1 -> G/1(m), C/1(m), M/1(m)
  "u "/1 -> Product/2
  Product/1 -> Add2/1
  M/1(y) -> Product/1
  qd/1 -> C/4(qd)
  q/1 -> G/2(q), C/3(q), M/3(q)
  Add2/1 -> "tau "/1
  C/1(y) -> Add2/2
  G/1(y) -> Add2/3

== matlab function sliding_controller2/Controller/F->tau1/Subsystem/MATLAB Function ==
  data: q input; y output
function y = fcn(q)

l1 = 0.3240;
y = [-l1*sin(q(1)), 0; l1*cos(q(1)), 0 ];


end

== matlab function sliding_controller2/Controller/F->tau1/Subsystem/MATLAB Function1 ==
  data: q input; y output
function y = fcn(q)

    l1 = 0.3240;
    l2 = 0.3900;
    y = [-l1*sin(q(1))-l2*sin(q(1)+q(2)), l1*cos(q(1)) + l2*sin(q(1)+q(2));...
         -l2*sin(q(1)+q(2)), l2*cos(q(1)+q(2))];
     
end

== matlab function sliding_controller2/Controller/F->tau1/Subsystem1/MATLAB Function ==
  data: q input; y output
function y = fcn(q)

l1 = 0.3240;
y = [-l1*sin(q(1)), 0; l1*cos(q(1)), 0 ];


end

== matlab function sliding_controller2/Controller/F->tau1/Subsystem1/MATLAB Function1 ==
  data: q input; y output
function y = fcn(q)

    l1 = 0.3240;
    l2 = 0.3900;
    y = [-l1*sin(q(1))-l2*sin(q(1)+q(2)), l1*cos(q(1)) + l2*sin(q(1)+q(2));...
         -l2*sin(q(1)+q(2)), l2*cos(q(1)+q(2))];
     
end

== matlab function sliding_controller2/Controller/human msg ==
  data: blankMsg input; msg output Bus: SL_Bus_sliding_controller2_sensor_msgs_JointState
function msg = stringArrayAssign(blankMsg)
% stringArrayAssign - Assign a string array in a ROS message
%
%  blankMsg (input): A bus for a 'sensor_msgs/JointState' message. This is 
%      used to initialize the output.
%  msg (output): A bus for a 'sensor_msgs/JointState' message message, with 
%      Name field set to a string array.
%
%   Copyright 2015 The MathWorks, Inc.

%#codegen

% Note: The datatype of 'msg' has been explicitly set to the appropriate 
% Simulink bus type ("SL_Bus_robotROSMessageUsageExample_sensor_msgs_JointState"). 
%
% If the model name is changed, the datatype needs to be changed as well:
%   1) Click "Edit Data" in the Editor toolstrip to open "Ports and Data Manager"
%   2) Select "msg". From the "Type" dropdown, select "--- Refresh data types ---"
%   3) Set datatype to "Bus: SL_Bus_<modelname>_sensor_msgs_JointState"

strArrayToAssign = {'LeftHip', 'LeftKnee', 'LeftAnkle', 'RightHip', 'RightKnee', 'RightAnkle', 'blanck'};
msg = blankMsg;

% Set the number of strings in the string array.
% msg (sensor_msgs/JointState) includes the following fields
%           Name : array of std_msgs/String (string array)
%   Name_SL_Info : struct with fields CurrentLength, ReceivedLength
numStringsInArray = length(strArrayToAssign);
msg.Name_SL_Info.CurrentLength = uint32(numStringsInArray);
msg.Velocity_SL_Info.CurrentLength = uint32(numStringsInArray);
msg.Position_SL_Info.CurrentLength = uint32(numStringsInArray);

% Set the individual strings in the array
for idx=1:numStringsInArray
    str = strArrayToAssign{idx};
    strLength = length(str);
    msg.Name(idx).Data(1:strLength) = uint8(str);
    msg.Name(idx).Data_SL_Info.CurrentLength = uint32(strLength);
end

== matlab function sliding_controller2/Controller/addmittance/MATLAB Function ==
  data: Kp0 input; Kn0 input; Bp0 input; Bn0 input; beta input; alpha input; Tid input; K output; Th input; qd input; B output
function [K,B] = fcn(Kp0, Kn0, Bp0, Bn0, beta, alpha,Tid, Th, qd)

Kp0 = diag(Kp0);
Kn0 = diag(Kn0);% [500 0; 0 500];
Bp0 = diag(Bp0);% [500 0; 0 500];
Bn0 =  diag(Bn0);%[500 0; 0 500];
beta_p = beta(1);
beta_n = beta(2);
alpha_p = alpha(1);
alpha_n = alpha(2);


intention = sign(Th) == sign(qd);
change = abs(Th/Tid);

K = eye(size(intention,1));
B = eye(size(intention,1));
count = 1;
my_intention = zeros(7,1);


for ii =  1:length(intention)
   if intention(ii)
        K(count,count) = Kp0(count,count) + beta_p*change(count);
        B(count,count) = Bp0(count,count) + alpha_p*change(count);
   else
       K(count,count) = Kn0(count,count) - beta_n*change(count);
       B(count,count) = Bn0(count,count) - alpha_n*change(count);
   end
   my_intention(count) = 0;
   count= count + 1;
   

end


end

== matlab function sliding_controller2/Controller/ interaction sping-damper/exo left ==
  data: q input; knee output; dknee output; qd input; ankle output; danke output
function [knee, dknee,ankle, danke]  = fcn(q, qd)


[knee, ankle, dknee, danke] = forward_kinimatics_leg(q,qd);
end

== matlab function sliding_controller2/Controller/ interaction sping-damper/exo right ==
  data: q input; knee output; dknee output; qd input; ankle output; danke output
function [knee, dknee,ankle, danke]  = fcn(q, qd)


[knee, ankle, dknee, danke] = forward_kinimatics_leg(q,qd);
end

== matlab function sliding_controller2/Controller/F->tau/Subsystem/MATLAB Function ==
  data: q input; y output
function y = fcn(q)

l1 = 0.3240;
y = [-l1*sin(q(1)), 0; l1*cos(q(1)), 0 ];


end

== matlab function sliding_controller2/Controller/F->tau/Subsystem/MATLAB Function1 ==
  data: q input; y output
function y = fcn(q)

    l1 = 0.3240;
    l2 = 0.3900;
    y = [-l1*sin(q(1))-l2*sin(q(1)+q(2)), l1*cos(q(1)) + l2*sin(q(1)+q(2));...
         -l2*sin(q(1)+q(2)), l2*cos(q(1)+q(2))];
     
end

== matlab function sliding_controller2/Controller/ interaction sping-damper/human left ==
  data: q input; knee output; dknee output; qd input; ankle output; danke output
function [knee, dknee,ankle, danke]  = fcn(q, qd)


[knee, ankle, dknee, danke] = forward_kinimatics_leg(q,qd);
end

== matlab function sliding_controller2/MATLAB Function - String Array Assign ==
  data: blankMsg input; msg output Bus: SL_Bus_sliding_controller2_RBDLInverseDynamicsReques_b5z6ex
function msg = stringArrayAssign(blankMsg)
% stringArrayAssign - Assign a string array in a ROS message
%
%  blankMsg (input): A bus for a 'sensor_msgs/JointState' message. This is 
%      used to initialize the output.
%  msg (output): A bus for a 'sensor_msgs/JointState' message message, with 
%      Name field set to a string array.
%
%   Copyright 2015 The MathWorks, Inc.

%#codegen

% Note: The datatype of 'msg' has been explicitly set to the appropriate 
% Simulink bus type ("SL_Bus_robotROSMessageUsageExample_sensor_msgs_JointState"). 
%
% If the model name is changed, the datatype needs to be changed as well:
%   1) Click "Edit Data" in the Editor toolstrip to open "Ports and Data Manager"
%   2) Select "msg". From the "Type" dropdown, select "--- Refresh data types ---"
%   3) Set datatype to "Bus: SL_Bus_<modelname>_sensor_msgs_JointState"

strArrayToAssign = {'exo'};
msg = blankMsg;
name = 'exo';
strLength = length(name);
% Set the number of strings in the string array.
% msg (sensor_msgs/JointState) includes the following fields
%           Name : array of std_msgs/String (string array)
%   Name_SL_Info : struct with fields CurrentLength, ReceivedLength
numStringsInArray = length(strArrayToAssign);
msg.ModelName_SL_Info.CurrentLength = uint32(strLength); % uint32(numStringsInArray);

msg.ModelName(1:strLength) = uint8(name);
msg.Q_SL_Info.CurrentLength = uint32(7);
msg.Qd_SL_Info.CurrentLength = uint32(7);
msg.Qdd_SL_Info.CurrentLength = uint32(7);

% % Set the individual strings in the array
% for idx=1:numStringsInArray
%     str = strArrayToAssign{idx};
%     strLength = length(str);
%     msg.ModelName(idx).Data(1:strLength) = uint8(str);
%     msg.Name(idx).Data_SL_Info.CurrentLength = uint32(strLength);
% end

== matlab function sliding_controller2/Controller/human controller/inv model 2/C ==
  data: m input; l input; q input; y output; qd input
function y = fcn(m, l, q, qd)



y = C(m, l, q, qd); % [m(2)*l(2)*qd(2)*qd(2)*sin(q(1)-q(2)); -m(2)*l(1)*qd(1)*qd(1)*sin(q(1)-q(2))];

== matlab function sliding_controller2/Controller/human controller/inv model 2/G ==
  data: m input; q input; y output
function y = fcn(m, q)
 y =  G(m,q);
end

== matlab function sliding_controller2/Controller/human controller/inv model 2/M ==
  data: m input; l input; q input; y output
function y = fcn(m, l, q)

y = M(m,l,q); % pinv([ (m(1)+m(2)) *l(1), m(2)*l(2)*cos(q(1)-q(2)); m(2)* l(1)*cos(q(1)-q(2)), m(2)*l(2)] );

end

== matlab function sliding_controller2/exo msg ==
  data: blankMsg input; msg output Bus: SL_Bus_sliding_controller2_sensor_msgs_JointState
function msg = stringArrayAssign(blankMsg)
% stringArrayAssign - Assign a string array in a ROS message
%
%  blankMsg (input): A bus for a 'sensor_msgs/JointState' message. This is 
%      used to initialize the output.
%  msg (output): A bus for a 'sensor_msgs/JointState' message message, with 
%      Name field set to a string array.
%
%   Copyright 2015 The MathWorks, Inc.

%#codegen

% Note: The datatype of 'msg' has been explicitly set to the appropriate 
% Simulink bus type ("SL_Bus_robotROSMessageUsageExample_sensor_msgs_JointState"). 
%
% If the model name is changed, the datatype needs to be changed as well:
%   1) Click "Edit Data" in the Editor toolstrip to open "Ports and Data Manager"
%   2) Select "msg". From the "Type" dropdown, select "--- Refresh data types ---"
%   3) Set datatype to "Bus: SL_Bus_<modelname>_sensor_msgs_JointState"

strArrayToAssign = {'LeftExoHip', 'LeftExoKnee', 'LeftExoAnkle', 'RightExoHip', 'RightExoKnee', 'RightExoAnkle', 'Crutches'};
msg = blankMsg;

% Set the number of strings in the string array.
% msg (sensor_msgs/JointState) includes the following fields
%           Name : array of std_msgs/String (string array)
%   Name_SL_Info : struct with fields CurrentLength, ReceivedLength
numStringsInArray = length(strArrayToAssign);
msg.Name_SL_Info.CurrentLength = uint32(numStringsInArray);
msg.Effort_SL_Info.CurrentLength = uint32(numStringsInArray);

% Set the individual strings in the array
for idx=1:numStringsInArray
    str = strArrayToAssign{idx};
    strLength = length(str);
    msg.Name(idx).Data(1:strLength) = uint8(str);
    msg.Name(idx).Data_SL_Info.CurrentLength = uint32(strLength);
end

== matlab function sliding_controller2/Controller/F->tau/Subsystem1/MATLAB Function ==
  data: q input; y output
function y = fcn(q)

l1 = 0.3240;
y = [-l1*sin(q(1)), 0; l1*cos(q(1)), 0 ];


end

== matlab function sliding_controller2/human msg ==
  data: blankMsg input; msg output Bus: SL_Bus_sliding_controller2_sensor_msgs_JointState
function msg = stringArrayAssign(blankMsg)
% stringArrayAssign - Assign a string array in a ROS message
%
%  blankMsg (input): A bus for a 'sensor_msgs/JointState' message. This is 
%      used to initialize the output.
%  msg (output): A bus for a 'sensor_msgs/JointState' message message, with 
%      Name field set to a string array.
%
%   Copyright 2015 The MathWorks, Inc.

%#codegen

% Note: The datatype of 'msg' has been explicitly set to the appropriate 
% Simulink bus type ("SL_Bus_robotROSMessageUsageExample_sensor_msgs_JointState"). 
%
% If the model name is changed, the datatype needs to be changed as well:
%   1) Click "Edit Data" in the Editor toolstrip to open "Ports and Data Manager"
%   2) Select "msg". From the "Type" dropdown, select "--- Refresh data types ---"
%   3) Set datatype to "Bus: SL_Bus_<modelname>_sensor_msgs_JointState"

strArrayToAssign = {'LeftHumanHip', 'LeftHumanKnee', 'LeftHumanAnkle', 'RightHumanHip', 'RightHumanKnee', 'RightHumanAnkle'};
msg = blankMsg;

% Set the number of strings in the string array.
% msg (sensor_msgs/JointState) includes the following fields
%           Name : array of std_msgs/String (string array)
%   Name_SL_Info : struct with fields CurrentLength, ReceivedLength
numStringsInArray = length(strArrayToAssign);
msg.Name_SL_Info.CurrentLength = uint32(numStringsInArray);
msg.Effort_SL_Info.CurrentLength = uint32(numStringsInArray);

% Set the individual strings in the array
for idx=1:numStringsInArray
    str = strArrayToAssign{idx};
    strLength = length(str);
    msg.Name(idx).Data(1:strLength) = uint8(str);
    msg.Name(idx).Data_SL_Info.CurrentLength = uint32(strLength);
end

== matlab function sliding_controller2/Controller/F->tau/Subsystem1/MATLAB Function1 ==
  data: q input; y output
function y = fcn(q)

    l1 = 0.3240;
    l2 = 0.3900;
    y = [-l1*sin(q(1))-l2*sin(q(1)+q(2)), l1*cos(q(1)) + l2*sin(q(1)+q(2));...
         -l2*sin(q(1)+q(2)), l2*cos(q(1)+q(2))];
     
end

== matlab function sliding_controller2/Controller/ interaction sping-damper/human right ==
  data: q input; knee output; dknee output; qd input; ankle output; danke output
function [knee, dknee,ankle, danke]  = fcn(q, qd)


[knee, ankle, dknee, danke] = forward_kinimatics_leg(q,qd);
end
